simulink model "sideslip_loop"  (R2019a)
settings: Solver=VariableStepAuto  StartTime=0.0  StopTime=1000  RelTol=1e-3
undefined symbols (not defined in the file or in its folder): AP, trans_func
settings Model: Creator=nikhil  LastModifiedBy=VTOL_HYD

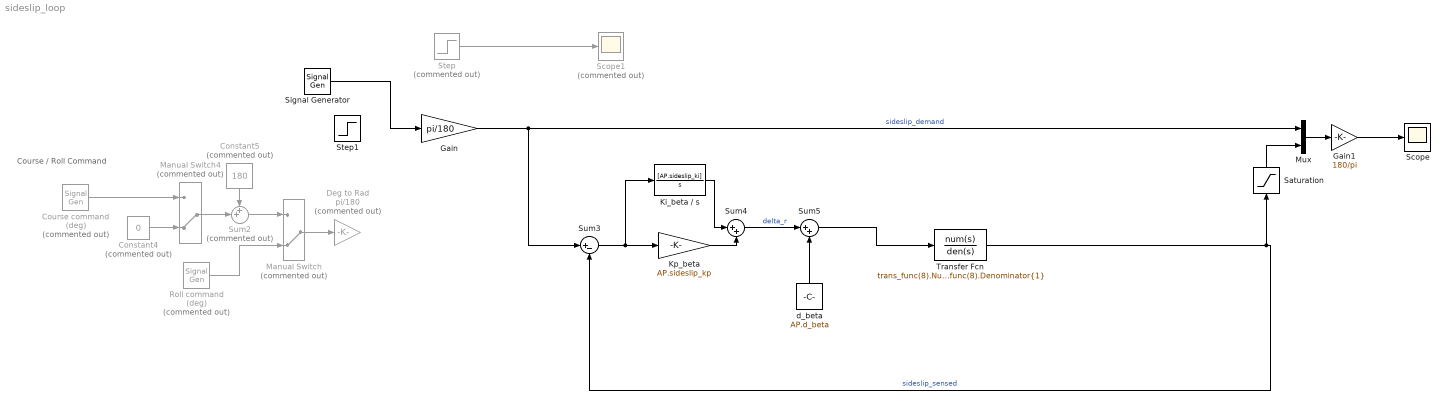
== system sideslip_loop ==
  note: Course / Roll Command
  Constant4 : Constant  Commented=on  Value=0
  Constant5 : Constant  Commented=on  Value=180
  Course command (deg) : SignalGenerator  Commented=on  WaveForm=square  Amplitude=45  Frequency=.02
  Deg to Rad : Gain  Commented=on  Gain=pi/180
  Gain : Gain  Gain=pi/180
  Gain1 : Gain  Gain=180/pi
  Ki_beta / s : TransferFcn  Numerator=[AP.sideslip_ki]  Denominator=[1 0]
  Kp_beta : Gain  Gain=AP.sideslip_kp
  Manual Switch : ManualSwitch  Commented=on  CurrentSetting=0
  Manual Switch4 : ManualSwitch  Commented=on  CurrentSetting=0
  Mux : Mux  Inputs=2
  Roll command (deg) : SignalGenerator  Commented=on  Amplitude=180  Frequency=0.1
  Saturation : Saturate  UpperLimit=3.14  LowerLimit=-3.14
  Scope : Scope
  Scope1 : Scope  Commented=on
  Signal Generator : SignalGenerator  WaveForm=square  Amplitude=25  Frequency=0.1  Units=rad/sec
  Step : Step  Commented=on  Time=8  After=25  SampleTime=0
  Step1 : Step  Time=20  After=25  SampleTime=0
  Sum2 : Sum  Commented=on  Inputs=++|
  Sum3 : Sum  Inputs=|+-
  Sum4 : Sum  Inputs=|++
  Sum5 : Sum  Inputs=|++
  Transfer Fcn : TransferFcn  Numerator=trans_func(8).Numerator{1}  Denominator=trans_func(8).Denominator{1}
  d_beta : Constant  Value=AP.d_beta
  wires:
  Course command (deg)/1 -> Manual Switch4/1
  Constant5/1 -> Sum2/1
  Manual Switch/1 -> Deg to Rad/1
  Manual Switch4/1 -> Sum2/2
  Sum2/1 -> Manual Switch/1
  Constant4/1 -> Manual Switch4/2
  Roll command (deg)/1 -> Manual Switch/2
  Gain/1 -> Sum3/1, Mux/1  "sideslip_demand"
  Transfer Fcn/1 -> Sum3/2, Saturation/1  "sideslip_sensed"
  Sum3/1 -> Ki_beta / s/1, Kp_beta/1
  Ki_beta / s/1 -> Sum4/1
  Kp_beta/1 -> Sum4/2
  Step/1 -> Scope1/1
  Saturation/1 -> Mux/2
  Mux/1 -> Gain1/1
  Gain1/1 -> Scope/1
  Sum5/1 -> Transfer Fcn/1
  d_beta/1 -> Sum5/2
  Sum4/1 -> Sum5/1  "delta_r"
  Signal Generator/1 -> Gain/1
